simulink library "Pipe_basic"  (Simulink 8.2)
settings: Solver=ode45  StartTime=0.0  StopTime=10.0  RelTol=1e-3
undefined symbols (not defined in the file): cond, cwall, d, l, nodes, t0, uloss
settings Model: Creator=drhf  LastModifiedBy=drhf

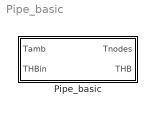
== system Pipe_basic ==
  Pipe_basic : Subsystem  mask(Pipe basic){vol=pi*(d/2)^2*l, L=l, uloss=uloss, effcond=cond, cwall=cwall, t0=t0, nodes=nodes}
      mask prompts: vol "Volume [m³]"; L "Length of pipe [m]"; uloss "Heat loss per pipe length [W/(m*K)]"; effcond "Effective conductivity of pipe wall [W/(m*K)]"; cwall "Capacity of pipewall per length [J/(m*K)]"; t0 "initial temperature [degree centigrade]"; nodes "number of nodes"
      mask help:
      | Multinode pipe with capacity. The flow is calculated by the upwind scheme heat conduction between nodes by central differences (Patankar 1980).
      | heat loss: u = conductivity / ( d_in * ln (d_out / d_in) )
      mask init:
      | nodes = max(nodes, 1);
      | vnode = max(vol,0.0001)/nodes;
      | lnode = max(L, 0.001)/nodes;
      | cnode = max(0.001,cwall)*L/vnode;
      | unode = uloss*lnode/vnode;
      | cond = effcond/(lnode*lnode);
      mask Help: web(fullfile(path_carnot('help'),'Pipe_basic.html'),'-helpbrowser')
      mask Display: plot(0,0,100,100,[24,27,27,24,75,80,80,75,24,20,20,24],[60,53,46,40,40,46,55,60,60,53,46,40])

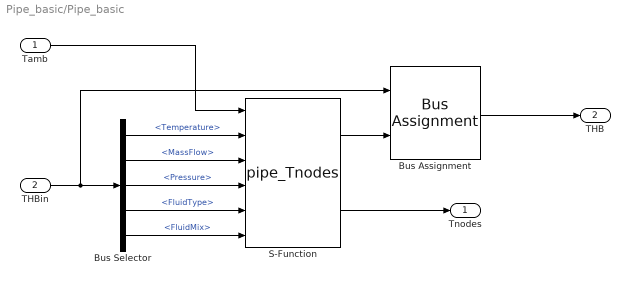
== system Pipe_basic/Pipe_basic ==
  Tamb : Inport
  THBin : Inport  Port=2
  Bus Assignment : BusAssignment  AssignedSignals=Temperature
  Bus Selector : BusSelector  OutputSignals=Temperature,MassFlow,Pressure,FluidType,FluidMix
  S-Function : S-Function  FunctionName=pipe_Tnodes  Parameters="vnode, lnode,  unode,  cond,  cnode,  t0, nodes"  EnableBusSupport=off
  Tnodes : Outport
  THB : Outport  Port=2
  wires:
  Bus Assignment/1 -> THB/1
  S-Function/2 -> Tnodes/1
  Bus Selector/5 -> S-Function/6  "<FluidMix>"
  Bus Selector/4 -> S-Function/5  "<FluidType>"
  Bus Selector/3 -> S-Function/4  "<Pressure>"
  Bus Selector/2 -> S-Function/3  "<MassFlow>"
  Bus Selector/1 -> S-Function/2  "<Temperature>"
  Tamb/1 -> S-Function/1
  S-Function/1 -> Bus Assignment/2
  THBin/1 -> Bus Selector/1, Bus Assignment/1
